simulink model "svpwm"  (R2021a)
settings: Solver=VariableStepAuto  StartTime=0.0  StopTime=10.0  RelTol=1e-3
undefined symbols (not defined in the file or in its folder): Tsc
libraries: eePwmGeneratorTwoLevel x1
settings Model: Creator=Sujit  LastModifiedBy=Sujit

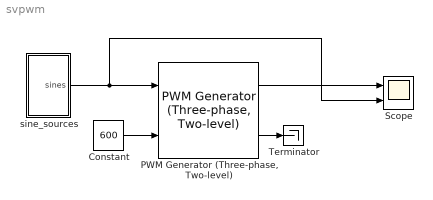
== system svpwm ==
  Constant : Constant  Value=600
  "PWM Generator (Three-phase, Two-level)" : eePwmGeneratorTwoLevel/PWM Generator (Three-phase, Two-level)  PWMMode=Continuous PWM (CPWM)  CPWMMode=SVM: space vector modulation  DPWMMode=60 DPWM: 60 degree discontinuous PWM  fsw=fs  Ts=Tsc
      settings: SourceProductBaseCode=PS
  Scope : Scope  NumInputPorts=2
  Terminator : Terminator
  sine_sources : Subsystem
  wires:
  sine_sources/1(sines) -> Scope/2, "PWM Generator (Three-phase, Two-level)"/1
  Constant/1 -> "PWM Generator (Three-phase, Two-level)"/2
  "PWM Generator (Three-phase, Two-level)"/1 -> Scope/1
  "PWM Generator (Three-phase, Two-level)"/2 -> Terminator/1

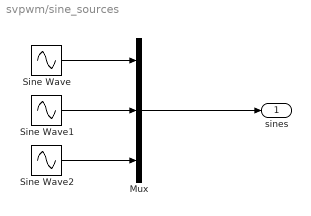
== system svpwm/sine_sources ==
  Mux : Mux  Inputs=3
  Sine Wave : Sin  Frequency=1257  SampleTime=0
  Sine Wave1 : Sin  Frequency=1257  Phase=(2*pi)/3  SampleTime=0
  Sine Wave2 : Sin  Frequency=1257  Phase=(4*pi)/3  SampleTime=0
  sines : Outport
  wires:
  Sine Wave1/1 -> Mux/2
  Sine Wave/1 -> Mux/1
  Mux/1 -> sines/1
  Sine Wave2/1 -> Mux/3
